simulink model "scattering"  (R2021a)
settings: Solver=FixedStepAuto  StartTime=0.0  StopTime=10  FixedStep=0.001  RelTol=1e-3
values from neighbouring files (symbols this model uses):
  B = 1    [scattering_params.m]    (also in scattering_params_vel.m)
  Be = 100    [scattering_params.m]    (also in scattering_params_vel.m = 15)
  Bh = 1.5    [scattering_params.m]    (also in scattering_params_vel.m = 70)
  Bs = 100    [scattering_params.m]    (also in scattering_params_vel.m = 5)
  Dh = 0.45    [scattering_params.m]    (also in scattering_params_vel.m = 10)
  Dm = 0    [scattering_params.m]    (also in scattering_params_vel.m)
  Ds = 0    [scattering_params.m]    (also in scattering_params_vel.m)
  Je = 0    [scattering_params.m]    (also in scattering_params_vel.m)
  Jh = 0.05    [scattering_params.m]    (also in scattering_params_vel.m)
  Ke = 200    [scattering_params.m]    (also in scattering_params_vel.m = 50)
  Kh = 1    [scattering_params.m]    (also in scattering_params_vel.m = 200)
  ki_s = 30    [scattering_params.m]
  kp_s = 750    [scattering_params.m]
  Ks = 20    [scattering_params.m]    (also in scattering_params_vel.m = 140)
  Mm = 0.5    [scattering_params.m]    (also in scattering_params_vel.m)
  Ms = 2    [scattering_params.m]    (also in scattering_params_vel.m)
  Ph = 2    [scattering_params.m]    (also in scattering_params_vel.m = 55)
  Ts = 0.001    [scattering_params.m]    (also in scattering_params_vel.m)
undefined symbols (not defined in the file or in its folder): tau
libraries: simulink x8
settings Model: Creator=anuj  LastModifiedBy=antoninoparisi
settings DebuggingCC: SFMachineParentedDataDiag=warning

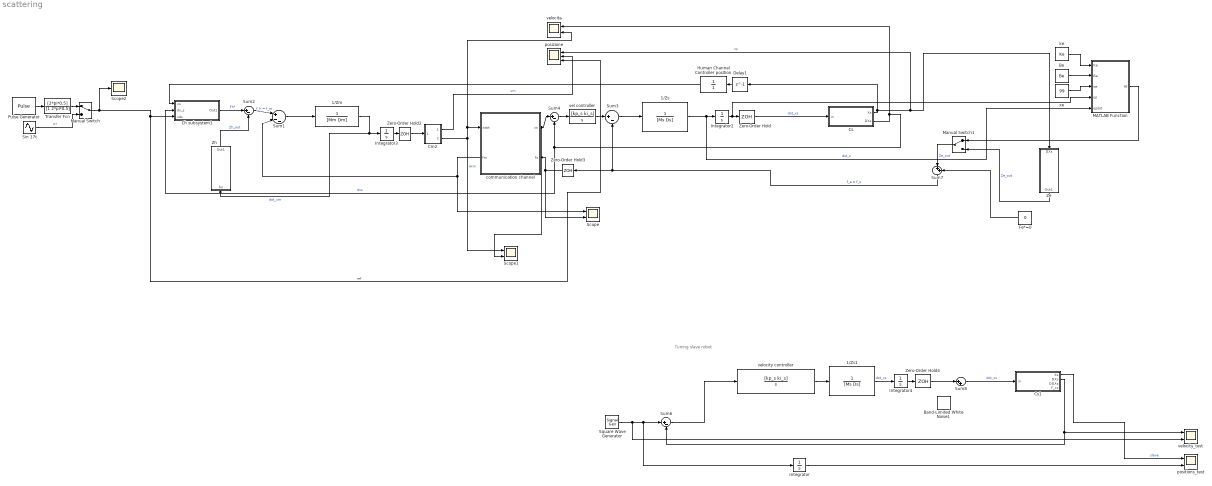
== system scattering ==
  note: Tuning slave robot
  1/Zm : TransferFcn  Denominator=[Mm Dm]
  1/Zs : TransferFcn  Denominator=[Ms Ds]
  1/Zs1 : TransferFcn  Denominator=[Ms Ds]
  Band-Limited White Noise1 : simulink/Sources/Band-Limited White Noise  Cov=[0.000001]  Ts=Ts  seed=[23341]
  Be : Constant  Value=Be
  Ch subsystem1 : Subsystem
  Cm2 : Subsystem
  Cs : Subsystem
  Cs1 : Subsystem
  Delay1 : Delay  DelayLength=1  SampleTime=Ts
  Fe*=0 : Constant  Value=0
  Human Channel Controller position : TransferFcn  Denominator=[1]
  Integrator{,2..4} (4 alike) : Integrator
  MATLAB Function : MATLAB Function  TreatAsAtomicUnit=on
  Manual Switch : ManualSwitch
  Manual Switch1 : ManualSwitch
  Pulse Generator : DiscretePulseGenerator  PulseType=Time based  Period=10  PulseWidth=50  PhaseDelay=1
  Scope : Scope  NumInputPorts=2
  Scope1 : Scope  NumInputPorts=2
  Scope2 : Scope
  Sin 17t : Sin  Amplitude=0.5  Frequency=2*pi*1  SampleTime=0
  Square Wave Generator : SignalGenerator  WaveForm=square  Units=rad/sec
  Sum1 : Sum  Inputs=|+--
  Sum{2..4,6} (4 alike) : Sum  Inputs=|+-
  Sum7 : Sum  Inputs=|++
  Sum8 : Sum  Inputs=|++
  Transfer Fcn : TransferFcn  Numerator=[2*pi*0.5]  Denominator=[1 2*pi*0.5]
  Ze : Subsystem
  Zero-Order Hold : ZeroOrderHold  SampleTime=-1
  Zero-Order Hold2 : ZeroOrderHold  SampleTime=-1
  Zero-Order Hold3 : ZeroOrderHold  SampleTime=Ts
  Zero-Order Hold4 : ZeroOrderHold  SampleTime=-1
  Zh : Subsystem
  communication channel : Subsystem
      settings: PortSchema="{\"entries\":[{\"content\":{\"sides\":[{\"content\":{\"connectorIds\":[\"In1\",\"Out2\"]},\"type\":\"ConnectorPlacement.EquallySpacedRectSide\",\"uuid\":\"e201856c-da4b-4980-a88b-c6c86de05881\"},{\"content\":{\"connectorIds\":[\"Out1\",\"In2\"],\"side\":\"RIGHT\"},\"type\":\"ConnectorPlacement.EquallySpacedRectSide\",\"uuid\":\"94e31da8-7242-4dd7-9573-e1ea0d94f21a\"},{\"content\":{\"connectorIds\":[],\"side\":\"TOP\"},\"type\":\"ConnectorPlacement.EquallySpacedRectSide\",\"uuid\":\"bf228117-dafc-454a-bb50-819d6ba8707f\"}]},\"type\":\"ConnectorPlacement.EquallySpacedConnector\",\"uuid\":\"7a0eb8a2-b25a-4eac-8153-08b01a29f1b4\"}],\"packageUris\":[\"http://schema.mathworks.com/mf0/Connector/R2020b\"],\"version\":\"1.0\"}"
  ke : Constant  Value=Ke
  positions_test : Scope  NumInputPorts=2
  posizione : Scope  NumInputPorts=3
  vel controller : TransferFcn  Numerator=[kp_s ki_s]  Denominator=[1 0]
  velocita : Scope  NumInputPorts=2
  velocity controller : TransferFcn  Numerator=[kp_s ki_s]  Denominator=[1 0]
  velocity_test : Scope  NumInputPorts=2
  xe : Constant  Value=99
  wires:
  Sum2/1 -> Sum1/1  "f_h = f_m"
  Manual Switch1/1 -> Sum7/1  "Ze_out"
  Ch subsystem1/1(Out1) -> Sum2/1  "Fh*"
  MATLAB Function/1(fE) -> Manual Switch1/1
  1/Zm/1 -> Integrator3/1, Zh/1(fm)  "dot_xm"
  Sum1/1 -> 1/Zm/1
  Human Channel Controller position/1 -> Ch subsystem1/1(xs)
  Be/1 -> MATLAB Function/2(Be)
  Cs/1(Xs) -> Delay1/1, posizione/1, Ze/1(DXs)  "xs"
  Fe*=0/1 -> Sum7/2
  xe/1 -> MATLAB Function/3(qe)
  ke/1 -> MATLAB Function/1(Ke)
  Manual Switch/1 -> posizione/3, Ch subsystem1/3(xds), Scope2/1  "ref"
  Zh/1(Out1) -> Sum2/2  "Zh_out"
  Ze/1(Out1) -> Manual Switch1/2  "Ze_out"
  Zero-Order Hold/1 -> Cs/1(in)  "dot_xs"
  Integrator2/1 -> MATLAB Function/4(qs), Zero-Order Hold/1
  Integrator3/1 -> Zero-Order Hold2/1
  Cm2/2(DXm) -> velocita/2, communication channel/1(xdot), Scope1/1  "dxm"
  Zero-Order Hold2/1 -> Cm2/1(In1)
  Sum3/1 -> 1/Zs/1
  Sum7/1 -> Zero-Order Hold3/1, Sum3/2  "f_e = f_s"
  Zero-Order Hold3/1 -> communication channel/2(fs), Scope/2
  vel controller/1 -> Sum3/1
  Sum4/1 -> vel controller/1
  communication channel/1(xs) -> Scope1/2, Sum4/1
  Cs/2(DXs) -> velocita/1, Sum4/2, Ch subsystem1/2(dx_s)  "dxs"
  Integrator4/1 -> Zero-Order Hold4/1
  Zero-Order Hold4/1 -> Sum8/1
  Sum8/1 -> Cs1/1(in)  "dot_xs"
  1/Zs1/1 -> Integrator4/1  "dot_xs"
  Cs1/1(Xs) -> positions_test/1  "slave"
  communication channel/2(fm) -> Scope/1, Sum1/2
  Sum6/1 -> velocity controller/1
  Square Wave Generator/1 -> velocity_test/2, Integrator/1, Sum6/1
  Cs1/2(DXs) -> velocity_test/1, Sum6/2
  Integrator/1 -> positions_test/2
  Cm2/1(Xm) -> posizione/2  "xm"
  1/Zs/1 -> MATLAB Function/5(qsdot), Integrator2/1  "dot_s"
  Delay1/1 -> Human Channel Controller position/1
  velocity controller/1 -> 1/Zs1/1
  Pulse Generator/1 -> Transfer Fcn/1
  Transfer Fcn/1 -> Manual Switch/1
  Sin 17t/1 -> Manual Switch/2  "F*"

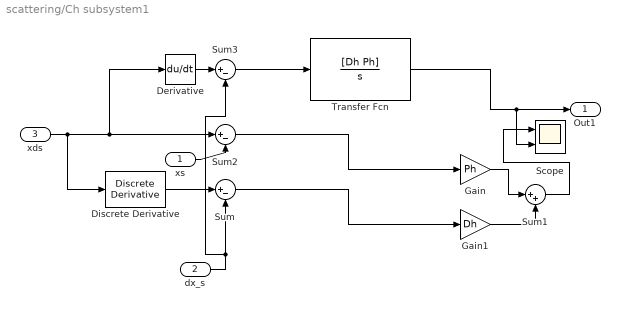
== system scattering/Ch subsystem1 ==
  xs : Inport
  dx_s : Inport  Port=2
  xds : Inport  Port=3
  Derivative : Derivative
  Discrete Derivative : simulink/Discrete/Discrete Derivative  gainval=1.0  ICPrevScaledInput=0.0  OutMin=[]  OutMax=[]  OutDataType=fixdt(1, 16)  OutScaling=2^-10  DoSatur=off
  Gain : Gain  Gain=Ph
  Gain1 : Gain  Gain=Dh
  Scope : Scope  NumInputPorts=2
  Sum : Sum  Inputs=|+-
  Sum1 : Sum  Inputs=|++
  Sum2 : Sum  Inputs=|+-
  Sum3 : Sum  Inputs=|+-
  Transfer Fcn : TransferFcn  Numerator=[Dh Ph]  Denominator=[1 0]
  Out1 : Outport
  wires:
  Gain1/1 -> Sum1/2
  Gain/1 -> Sum1/1
  xs/1 -> Sum2/2
  Discrete Derivative/1 -> Sum/1
  Sum/1 -> Gain1/1
  Sum2/1 -> Gain/1
  xds/1 -> Derivative/1, Sum2/1, Discrete Derivative/1
  dx_s/1 -> Sum3/2, Sum/2
  Derivative/1 -> Sum3/1
  Sum3/1 -> Transfer Fcn/1
  Transfer Fcn/1 -> Scope/2, Out1/1
  Sum1/1 -> Scope/1

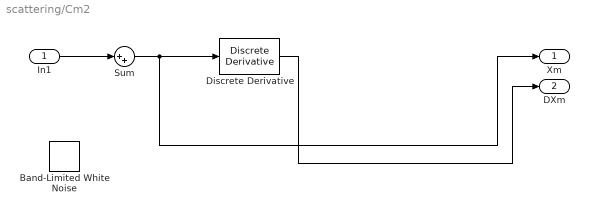
== system scattering/Cm2 ==
  In1 : Inport
  Band-Limited White Noise : simulink/Sources/Band-Limited White Noise  Cov=[0.0000001]  Ts=Ts  seed=[23341]
  Discrete Derivative : simulink/Discrete/Discrete Derivative  gainval=1.0  ICPrevScaledInput=0.0  OutMin=[]  OutMax=[]  OutDataType=fixdt(1, 16)  OutScaling=2^-10  DoSatur=off
  Sum : Sum  Inputs=|++
  Xm : Outport
  DXm : Outport  Port=2
  wires:
  Sum/1 -> Xm/1, Discrete Derivative/1
  Discrete Derivative/1 -> DXm/1
  In1/1 -> Sum/1

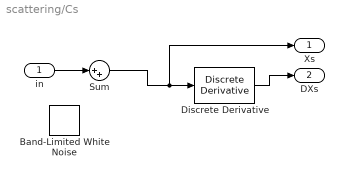
== system scattering/Cs ==
  in : Inport
  Band-Limited White Noise : simulink/Sources/Band-Limited White Noise  Cov=[0.000001]  Ts=Ts  seed=[23341]
  Discrete Derivative : simulink/Discrete/Discrete Derivative  gainval=1.0  ICPrevScaledInput=0.0  OutMin=[]  OutMax=[]  OutDataType=fixdt(1, 16)  OutScaling=2^-10  DoSatur=off
  Sum : Sum  Inputs=|++
  Xs : Outport
  DXs : Outport  Port=2
  wires:
  Discrete Derivative/1 -> DXs/1
  in/1 -> Sum/1
  Sum/1 -> Xs/1, Discrete Derivative/1

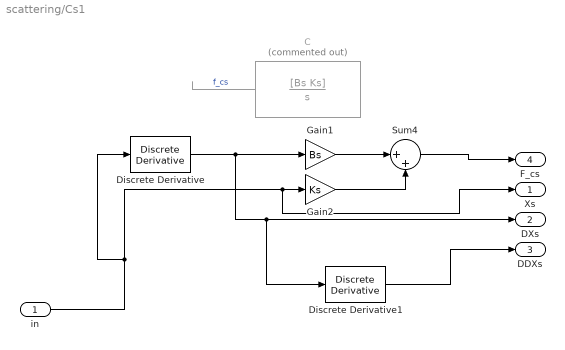
== system scattering/Cs1 ==
  in : Inport
  C : TransferFcn  Commented=on  Numerator=[Bs Ks]  Denominator=[1 0]
  Discrete Derivative : simulink/Discrete/Discrete Derivative  gainval=1.0  ICPrevScaledInput=0.0  OutMin=[]  OutMax=[]  OutDataType=fixdt(1, 16)  OutScaling=2^-10  DoSatur=off
  Discrete Derivative1 : simulink/Discrete/Discrete Derivative  gainval=1.0  ICPrevScaledInput=0.0  OutMin=[]  OutMax=[]  OutDataType=fixdt(1, 16)  OutScaling=2^-10  DoSatur=off
  Gain1 : Gain  Gain=Bs
  Gain2 : Gain  Gain=Ks
  Sum4 : Sum  Inputs=|++
  Xs : Outport
  DXs : Outport  Port=2
  DDXs : Outport  Port=3
  F_cs : Outport  Port=4
  wires:
  Sum4/1 -> F_cs/1
  Gain1/1 -> Sum4/1
  in/1 -> Xs/1, Gain2/1, Discrete Derivative/1
  Gain2/1 -> Sum4/2
  C/1 -> ?  "f_cs"
  Discrete Derivative/1 -> Discrete Derivative1/1, DXs/1, Gain1/1
  Discrete Derivative1/1 -> DDXs/1

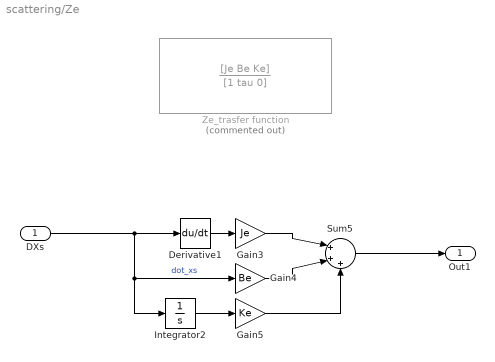
== system scattering/Ze ==
  DXs : Inport
  Derivative1 : Derivative
  Gain3 : Gain  Gain=Je
  Gain4 : Gain  Gain=Be
  Gain5 : Gain  Gain=Ke
  Integrator2 : Integrator
  Sum5 : Sum  Inputs=|+++
  Ze_trasfer function : TransferFcn  Commented=on  Numerator=[Je Be Ke]  Denominator=[1 tau 0]
  Out1 : Outport
  wires:
  Gain4/1 -> Sum5/2
  Gain3/1 -> Sum5/1
  Gain5/1 -> Sum5/3
  Sum5/1 -> Out1/1
  Integrator2/1 -> Gain5/1
  DXs/1 -> Integrator2/1, Gain4/1, Derivative1/1  "dot_xs"
  Derivative1/1 -> Gain3/1

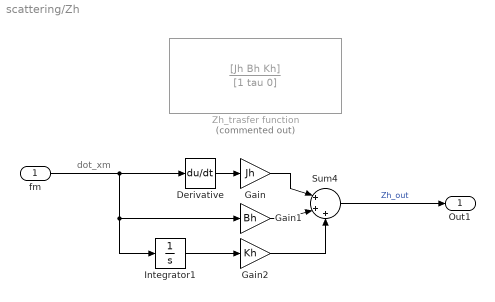
== system scattering/Zh ==
  note: dot_xm
  fm : Inport
  Derivative : Derivative
  Gain : Gain  Gain=Jh
  Gain1 : Gain  Gain=Bh
  Gain2 : Gain  Gain=Kh
  Integrator1 : Integrator
  Sum4 : Sum  Inputs=|+++
  Zh_trasfer function : TransferFcn  Commented=on  Numerator=[Jh Bh Kh]  Denominator=[1 tau 0]
  Out1 : Outport
  wires:
  Derivative/1 -> Gain/1
  Integrator1/1 -> Gain2/1
  Gain2/1 -> Sum4/3
  Gain1/1 -> Sum4/2
  Gain/1 -> Sum4/1
  Sum4/1 -> Out1/1  "Zh_out"
  fm/1 -> Gain1/1, Integrator1/1, Derivative/1

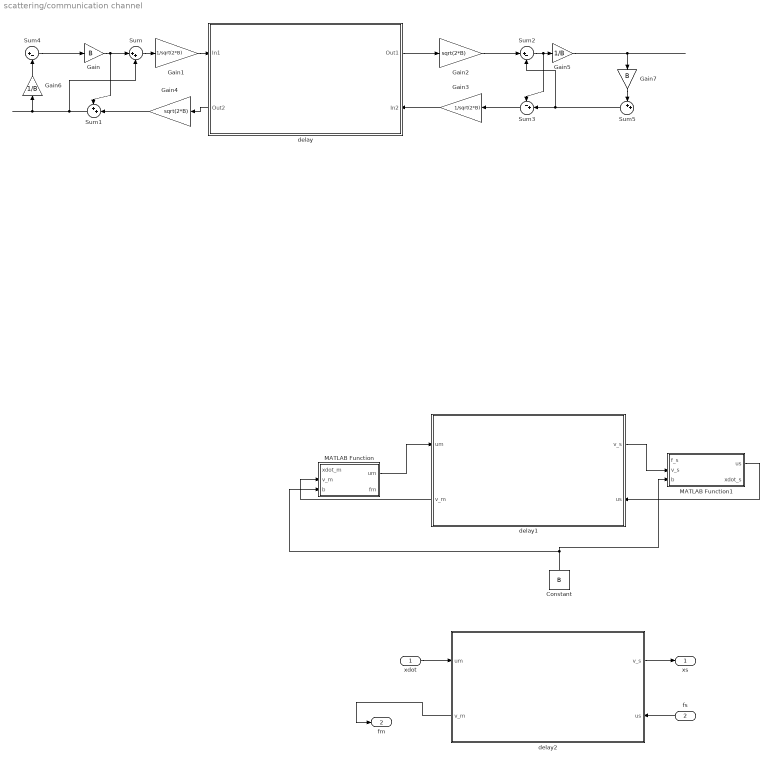
== system scattering/communication channel ==
  xdot : Inport
  fs : Inport  Port=2
  Constant : Constant  Value=B
  Gain : Gain  Gain=B
  Gain1 : Gain  Gain=1/sqrt(2*B)
  Gain2 : Gain  Gain=sqrt(2*B)
  Gain3 : Gain  Gain=1/sqrt(2*B)
  Gain4 : Gain  Gain=sqrt(2*B)
  Gain5 : Gain  Gain=1/B
  Gain6 : Gain  Gain=1/B
  Gain7 : Gain  Gain=B
  MATLAB Function : MATLAB Function  TreatAsAtomicUnit=on
  MATLAB Function1 : MATLAB Function  TreatAsAtomicUnit=on
  Sum : Sum  Inputs=|++
  Sum1 : Sum  Inputs=++|
  Sum2 : Sum  Inputs=|+-
  Sum3 : Sum  Inputs=-+|
  Sum4 : Sum  Inputs=|+-
  Sum5 : Sum  Inputs=++|
  delay : Subsystem
      settings: PortSchema="{\"entries\":[{\"content\":{\"sides\":[{\"content\":{\"connectorIds\":[\"In1\",\"Out2\"]},\"type\":\"ConnectorPlacement.EquallySpacedRectSide\",\"uuid\":\"e201856c-da4b-4980-a88b-c6c86de05881\"},{\"content\":{\"connectorIds\":[\"Out1\",\"In2\"],\"side\":\"RIGHT\"},\"type\":\"ConnectorPlacement.EquallySpacedRectSide\",\"uuid\":\"94e31da8-7242-4dd7-9573-e1ea0d94f21a\"},{\"content\":{\"connectorIds\":[],\"side\":\"TOP\"},\"type\":\"ConnectorPlacement.EquallySpacedRectSide\",\"uuid\":\"bf228117-dafc-454a-bb50-819d6ba8707f\"}]},\"type\":\"ConnectorPlacement.EquallySpacedConnector\",\"uuid\":\"7a0eb8a2-b25a-4eac-8153-08b01a29f1b4\"}],\"packageUris\":[\"http://schema.mathworks.com/mf0/Connector/R2020b\"],\"version\":\"1.0\"}"
  delay1 : Subsystem
      settings: PortSchema="{\"entries\":[{\"content\":{\"sides\":[{\"content\":{\"connectorIds\":[\"In1\",\"Out2\"]},\"type\":\"ConnectorPlacement.EquallySpacedRectSide\",\"uuid\":\"e201856c-da4b-4980-a88b-c6c86de05881\"},{\"content\":{\"connectorIds\":[\"Out1\",\"In2\"],\"side\":\"RIGHT\"},\"type\":\"ConnectorPlacement.EquallySpacedRectSide\",\"uuid\":\"94e31da8-7242-4dd7-9573-e1ea0d94f21a\"},{\"content\":{\"connectorIds\":[],\"side\":\"TOP\"},\"type\":\"ConnectorPlacement.EquallySpacedRectSide\",\"uuid\":\"bf228117-dafc-454a-bb50-819d6ba8707f\"}]},\"type\":\"ConnectorPlacement.EquallySpacedConnector\",\"uuid\":\"7a0eb8a2-b25a-4eac-8153-08b01a29f1b4\"}],\"packageUris\":[\"http://schema.mathworks.com/mf0/Connector/R2020b\"],\"version\":\"1.0\"}"
  delay2 : Subsystem
      settings: PortSchema="{\"entries\":[{\"content\":{\"sides\":[{\"content\":{\"connectorIds\":[\"In1\",\"Out2\"]},\"type\":\"ConnectorPlacement.EquallySpacedRectSide\",\"uuid\":\"e201856c-da4b-4980-a88b-c6c86de05881\"},{\"content\":{\"connectorIds\":[\"Out1\",\"In2\"],\"side\":\"RIGHT\"},\"type\":\"ConnectorPlacement.EquallySpacedRectSide\",\"uuid\":\"94e31da8-7242-4dd7-9573-e1ea0d94f21a\"},{\"content\":{\"connectorIds\":[],\"side\":\"TOP\"},\"type\":\"ConnectorPlacement.EquallySpacedRectSide\",\"uuid\":\"bf228117-dafc-454a-bb50-819d6ba8707f\"}]},\"type\":\"ConnectorPlacement.EquallySpacedConnector\",\"uuid\":\"7a0eb8a2-b25a-4eac-8153-08b01a29f1b4\"}],\"packageUris\":[\"http://schema.mathworks.com/mf0/Connector/R2020b\"],\"version\":\"1.0\"}"
  xs : Outport
  fm : Outport  Port=2
  wires:
  Constant/1 -> MATLAB Function/3(b), MATLAB Function1/3(b)
  MATLAB Function/1(um) -> delay1/1(um)
  delay1/1(v_s) -> MATLAB Function1/2(v_s)
  MATLAB Function1/1(us) -> delay1/2(us)
  Sum1/1 -> Sum/2, Gain6/1
  Sum4/1 -> Gain/1
  ? -> Sum4/1
  Gain5/1 -> Gain7/1
  Sum5/1 -> Sum3/2, Sum2/2
  Gain/1 -> Sum1/1, Sum/1
  Sum/1 -> Gain1/1
  Gain1/1 -> delay/1(In1)
  delay/2(Out2) -> Gain4/1
  Sum3/1 -> Gain3/1
  Gain6/1 -> Sum4/2
  Gain2/1 -> Sum2/1
  Gain4/1 -> Sum1/2
  delay/1(Out1) -> Gain2/1
  ? -> Sum5/2
  Gain3/1 -> delay/2(In2)
  Gain7/1 -> Sum5/1
  Sum2/1 -> Sum3/1, Gain5/1
  delay1/2(v_m) -> MATLAB Function/2(v_m)
  delay2/2(v_m) -> fm/1
  xdot/1 -> delay2/1(um)
  delay2/1(v_s) -> xs/1
  fs/1 -> delay2/2(us)

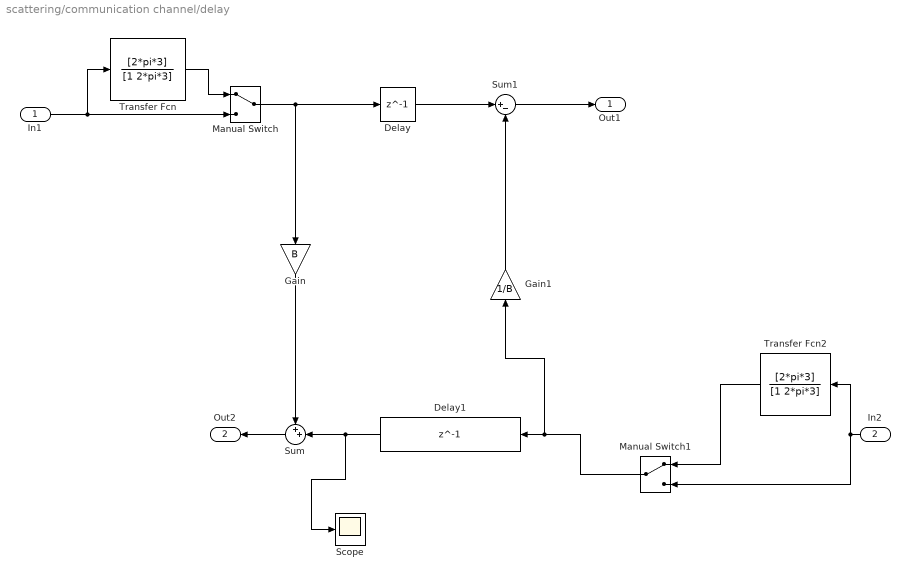
== system scattering/communication channel/delay ==
  In1 : Inport
  In2 : Inport  Port=2
  Delay : Delay  DelayLength=1  InitialCondition=0
  Delay1 : Delay  DelayLength=1  InitialCondition=0
  Gain : Gain  Gain=B
  Gain1 : Gain  Gain=1/B
  Manual Switch : ManualSwitch
  Manual Switch1 : ManualSwitch
  Scope : Scope
  Sum : Sum  Inputs=++|
  Sum1 : Sum  Inputs=|+-
  Transfer Fcn : TransferFcn  Numerator=[2*pi*3]  Denominator=[1 2*pi*3]
  Transfer Fcn2 : TransferFcn  Numerator=[2*pi*3]  Denominator=[1 2*pi*3]
  Out1 : Outport
  Out2 : Outport  Port=2
  wires:
  Sum/1 -> Out2/1
  Gain/1 -> Sum/1
  Gain1/1 -> Sum1/2
  Sum1/1 -> Out1/1
  Delay/1 -> Sum1/1
  Delay1/1 -> Scope/1, Sum/2
  In1/1 -> Transfer Fcn/1, Manual Switch/2
  Transfer Fcn/1 -> Manual Switch/1
  Manual Switch/1 -> Gain/1, Delay/1
  Transfer Fcn2/1 -> Manual Switch1/1
  In2/1 -> Transfer Fcn2/1, Manual Switch1/2
  Manual Switch1/1 -> Gain1/1, Delay1/1

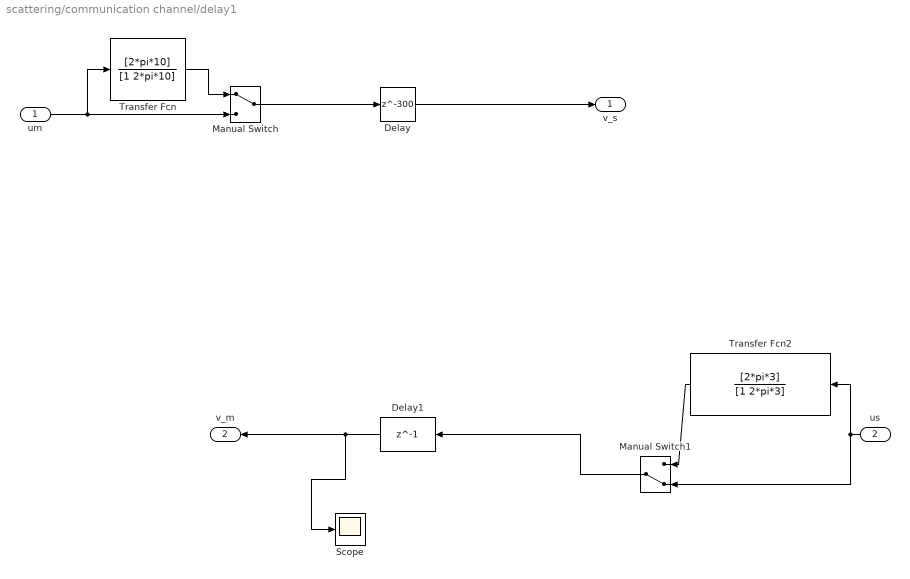
== system scattering/communication channel/delay1 ==
  um : Inport
  us : Inport  Port=2
  Delay : Delay  DelayLength=300  InitialCondition=0  SampleTime=Ts
  Delay1 : Delay  DelayLength=1  InitialCondition=0  SampleTime=Ts
  Manual Switch : ManualSwitch
  Manual Switch1 : ManualSwitch  CurrentSetting=0
  Scope : Scope
  Transfer Fcn : TransferFcn  Numerator=[2*pi*10]  Denominator=[1 2*pi*10]
  Transfer Fcn2 : TransferFcn  Numerator=[2*pi*3]  Denominator=[1 2*pi*3]
  v_s : Outport
  v_m : Outport  Port=2
  wires:
  Delay1/1 -> v_m/1, Scope/1
  Delay/1 -> v_s/1
  um/1 -> Transfer Fcn/1, Manual Switch/2
  Transfer Fcn/1 -> Manual Switch/1
  Manual Switch/1 -> Delay/1
  Transfer Fcn2/1 -> Manual Switch1/1
  us/1 -> Transfer Fcn2/1, Manual Switch1/2
  Manual Switch1/1 -> Delay1/1

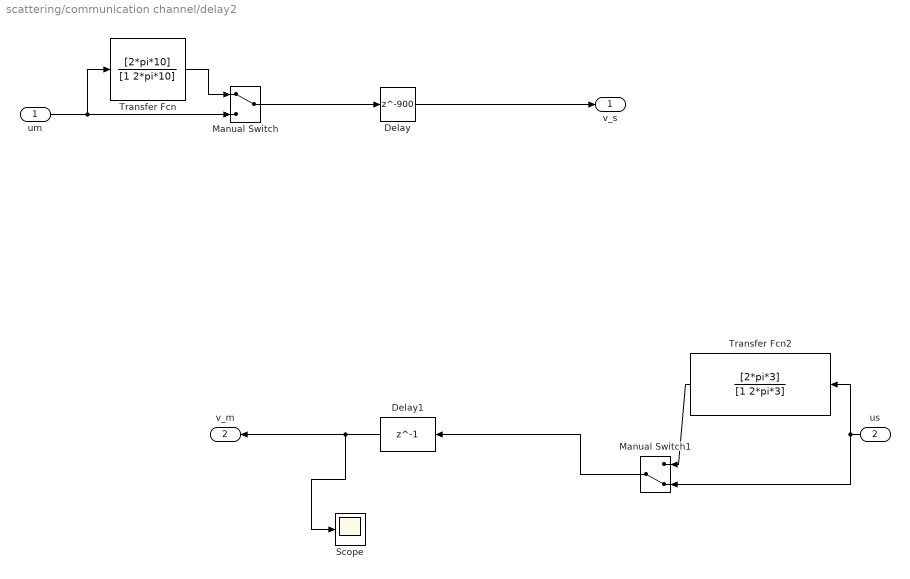
== system scattering/communication channel/delay2 ==
  um : Inport
  us : Inport  Port=2
  Delay : Delay  DelayLength=900  InitialCondition=0  SampleTime=Ts
  Delay1 : Delay  DelayLength=1  InitialCondition=0  SampleTime=Ts
  Manual Switch : ManualSwitch
  Manual Switch1 : ManualSwitch  CurrentSetting=0
  Scope : Scope
  Transfer Fcn : TransferFcn  Numerator=[2*pi*10]  Denominator=[1 2*pi*10]
  Transfer Fcn2 : TransferFcn  Numerator=[2*pi*3]  Denominator=[1 2*pi*3]
  v_s : Outport
  v_m : Outport  Port=2
  wires:
  Delay1/1 -> v_m/1, Scope/1
  Delay/1 -> v_s/1
  um/1 -> Transfer Fcn/1, Manual Switch/2
  Transfer Fcn/1 -> Manual Switch/1
  Manual Switch/1 -> Delay/1
  Transfer Fcn2/1 -> Manual Switch1/1
  us/1 -> Transfer Fcn2/1, Manual Switch1/2
  Manual Switch1/1 -> Delay1/1

== matlab function scattering/communication channel/MATLAB Function ==
  data: xdot_m input; v_m input; um output; b input; fm output
function [um,fm] = fcn(xdot_m,v_m,b)
% anti vibr
um = sqrt(b/2)*xdot_m;
fm = b/2*xdot_m + sqrt(b/2)*v_m;


um = sqrt(2*b)*xdot_m + v_m;
fm = b*xdot_m + sqrt(2*b)*v_m;
end

== matlab function scattering/MATLAB Function ==
  data: Ke input; fE output; Be input; qe input; qs input; qsdot input
function fE = environment(Ke, Be, qe, qs, qsdot)
    if qs > qe
        fE = Ke * (qs - qe) + Be * qsdot;
    else
        fE = 0;
    end
end

== matlab function scattering/communication channel/MATLAB Function1 ==
  data: f_s input; v_s input; us output; b input; xdot_s output
function [us,xdot_s] = fcn(f_s,v_s,b)

us = 1/sqrt(2*b)*f_s;
xdot_s = -0.5*b*f_s + 1/sqrt(2*b)*v_s;


us = sqrt(2/b)*f_s - v_s;
xdot_s = -1/b*(f_s - sqrt(2*b)*v_s);
